simulink model "ex_3_7_simul"  (R2025b)
settings: Solver=VariableStepAuto  StartTime=0.0  StopTime=30  MaxStep=0.1  RelTol=1e-3
settings Model: Creator=konstantin  LastModifiedBy=konstantin

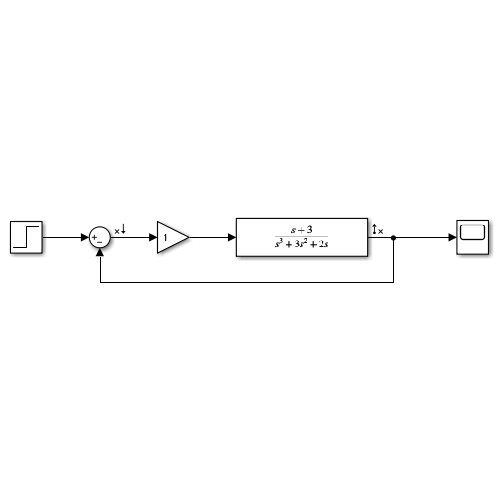
[thumbnail: Simulink's stored preview of the top-level diagram]
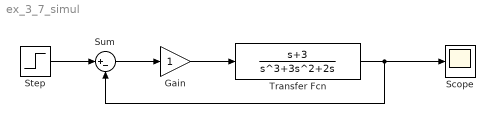
== system ex_3_7_simul ==
  Gain : Gain
  Scope : Scope
      settings: ActiveDisplayYMinimum=-0.16549529036847202  ActiveDisplayYMaximum=1.4894576133162485
  Step : Step  SampleTime=0
  Sum : Sum  Inputs=|+-
  Transfer Fcn : TransferFcn  Numerator=[1 3]  Denominator=[1 3 2 0]
  wires:
  Gain/1 -> Transfer Fcn/1
  Sum/1 -> Gain/1
  Transfer Fcn/1 -> Scope/1, Sum/2
  Step/1 -> Sum/1
